simulink model "BothOptimizedNew"  (R2024b)
settings: Solver=FixedStepAuto  StartTime=0.0  StopTime=10.0  RelTol=1e-3  EnableMultiTasking=on
undefined symbols (not defined in the file or in its folder): samplingTime
settings Model: STM32="{\"DigitalPortWrite\":[{\"ID\":\"MicroMouseTemplate:84:3\"},{\"ID\":\"MicroMouseTemplate:84:4\"},{\"ID\":\"MicroMouseTemplate:84:5\"},{\"ID\":\"MicroMouseTemplate:84:6\"},{\"ID\":\"MicroMouseTemplate:84:7\"},{\"ID\":\"MicroMouseTemplate:84:8\"},{\"ID\":\"MicroMouseTemplate:84:9\"},{\"ID\":\"MicroMouseTemplate:84:10\"},{\"ID\":\"MicroMouseTemplate:160:19\"},{\"ID\":\"MicroMouseTemplate:2479:4\"},{\"ID\":\"MicroMouseTemplate:2479:6\"},{\"ID\":\"MicroMouseTemplate:2479:7\"},{\"ID\":\"MicroMouseTemplate:2479:8\"},{\"ID\":\"MicroMouseTemplate2:160:19\"},{\"ID\":\"MicroMouseTemplate2:2479:4\"},{\"ID\":\"MicroMouseTemplate2:2479:6\"},{\"ID\":\"MicroMouseTemplate2:2479:7\"},{\"ID\":\"MicroMouseTemplate2:2479:8\"},{\"ID\":\"MicroMouseTemplate2:84:3\"},{\"ID\":\"MicroMouseTemplate2:84:4\"},{\"ID\":\"MicroMouseTemplate2:84:5\"},{\"ID\":\"MicroMouseTemplate2:84:6\"},{\"ID\":\"MicroMouseTemplate2:84:7\"},{\"ID\":\"MicroMouseTemplate2:84:8\"},{\"ID\":\"MicroMouseTemplate2:84:9\"},{\"ID\":\"MicroMouseTemplate2:84:10\"},{\"ID\":\"MicroMouseTemplateTest:160:19\"},{\"ID\":\"MicroMouseTemplateTest:2479:4\"},{\"ID\":\"MicroMouseTemplateTest:2479:6\"},{\"ID\":\"MicroMouseTemplateTest:2479:7\"},{\"ID\":\"MicroMouseTemplateTest:2479:8\"},{\"ID\":\"MicroMouseTemplateTest:84:3\"},{\"ID\":\"MicroMouseTemplateTest:84:4\"},{\"ID\":\"MicroMouseTemplateTest:84:5\"},{\"ID\":\"MicroMouseTemplateTest:84:6\"},{\"ID\":\"MicroMouseTemplateTest:84:7\"},{\"ID\":\"MicroMouseTemplateTest:84:8\"},{\"ID\":\"MicroMouseTemplateTest:84:9\"},{\"ID\":\"MicroMouseTemplateTest:84:10\"},{\"ID\":\"MicroMouseTemplateTest2:160:19\"},{\"ID\":\"MicroMouseTemplateTest2:2479:4\"},{\"ID\":\"MicroMouseTemplateTest2:2479:6\"},{\"ID\":\"MicroMouseTemplateTest2:2479:7\"},{\"ID\":\"MicroMouseTemplateTest2:2479:8\"},{\"ID\":\"MicroMouseTemplateTest2:84:3\"},{\"ID\":\"MicroMouseTemplateTest2:84:4\"},{\"ID\":\"MicroMouseTemplateTest2:84:5\"},{\"ID\":\"MicroMouseTemplateTest2:84:6\"},{\"ID\":\"MicroMouseTemplateTest2:84:7\"},{\"ID\":\"MicroMouseTemplateTest2:84:8\"},{\"ID\":\"MicroMouseTemplateTest2:84:9\"},{\"ID\":\"MicroMouseTemplateTest2:84:10\"},{\"ID\":\"HalfOptimized:84:10\"},{\"ID\":\"HalfOptimized:84:9\"},{\"ID\":\"HalfOptimized:84:8\"},{\"ID\":\"HalfOptimized:84:7\"},{\"ID\":\"HalfOptimized:84:6\"},{\"ID\":\"HalfOptimized:84:5\"},{\"ID\":\"HalfOptimized:84:4\"},{\"ID\":\"HalfOptimized:84:3\"},{\"ID\":\"HalfOptimized:160:19\"},{\"ID\":\"HalfOptimized:2479:4\"},{\"ID\":\"HalfOptimized:2479:6\"},{\"ID\":\"HalfOptimized:2479:7\"},{\"ID\":\"HalfOptimized:2479:8\"},{\"ID\":\"HalfOptimized4:84:3\"},{\"ID\":\"HalfOptimized4:84:4\"},{\"ID\":\"HalfOptimized4:84:5\"},{\"ID\":\"HalfOptimized4:84:6\"},{\"ID\":\"HalfOptimized4:84:7\"},{\"ID\":\"HalfOptimized4:84:8\"},{\"ID\":\"HalfOptimized4:84:9\"},{\"ID\":\"HalfOptimized4:84:10\"},{\"ID\":\"HalfOptimized4:160:19\"},{\"ID\":\"HalfOptimized4:2479:4\"},{\"ID\":\"HalfOptimized4:2479:6\"},{\"ID\":\"HalfOptimized4:2479:7\"},{\"ID\":\"HalfOptimized4:2479:8\"},{\"ID\":\"LeftOptimized4:84:3\"},{\"ID\":\"LeftOptimized4:84:4\"},{\"ID\":\"LeftOptimized4:84:5\"},{\"ID\":\"LeftOptimized4:84:6\"},{\"ID\":\"LeftOptimized4:84:7\"},{\"ID\":\"LeftOptimized4:84:8\"},{\"ID\":\"LeftOptimized4:84:9\"},{\"ID\":\"LeftOptimized4:84:10\"},{\"ID\":\"LeftOptimized4:160:19\"},{\"ID\":\"LeftOptimized4:2479:4\"},{\"ID\":\"LeftOptimized4:2479:6\"},{\"ID\":\"LeftOptimized4:2479:7\"},{\"ID\":\"LeftOptimized4:2479:8\"},{\"ID\":\"BothOptimizedNew:84:3\"},{\"ID\":\"BothOptimizedNew:84:4\"},{\"ID\":\"BothOptimizedNew:84:5\"},{\"ID\":\"BothOptimizedNew:84:6\"},{\"ID\":\"BothOptimizedNew:84:7\"},{\"ID\":\"BothOptimizedNew:84:8\"},{\"ID\":\"BothOptimizedNew:84:9\"},{\"ID\":\"BothOptimizedNew:84:10\"},{\"ID\":\"BothOptimizedNew:160:19\"},{\"ID\":\"BothOptimizedNew:2479:4\"},{\"ID\":\"BothOptimizedNew:2479:6\"},{\"ID\":\"BothOptimizedNew:2479:7\"},{\"ID\":\"BothOptimizedNew:2479:8\"}],\"PWMOutput\":[{\"ID\":\"MicroMouseTemplate:160:24\"},{\"ID\":\"MicroMouseTemplate:160:25\"},{\"ID\":\"MicroMouseTemplate2:160:24\"},{\"ID\":\"MicroMouseTemplate2:160:25\"},{\"ID\":\"MicroMouseTemplateTest:160:24\"},{\"ID\":\"MicroMouseTemplateTest:160:25\"},{\"ID\":\"MicroMouseTemplateTest2:160:24\"},{\"ID\":\"MicroMouseTemplateTest2:160:25\"},{\"ID\":\"HalfOptimized:160:24\"},{\"ID\":\"HalfOptimized:160:25\"},{\"ID\":\"HalfOptimized4:160:24\"},{\"ID\":\"HalfOptimized4:160:25\"},{\"ID\":\"LeftOptimized4:160:24\"},{\"ID\":\"LeftOptimized4:160:25\"},{\"ID\":\"BothOptimizedNew:160:24\"},{\"ID\":\"BothOptimizedNew:160:25\"}],\"AnalogInput\":[{\"ID\":\"MicroMouseTemplate:2357:1\"},{\"ID\":\"MicroMouseTemplate2:2357:1\"},{\"ID\":\"MicroMouseTemplateTest:2357:1\"},{\"ID\":\"MicroMouseTemplateTest2:2357:1\"},{\"ID\":\"HalfOptimized:2357:1\"},{\"ID\":\"HalfOptimized4:2357:1\"},{\"ID\":\"LeftOptimized4:2357:1\"},{\"ID\":\"BothOptimizedNew:2357:1\"}],\"DigitalPortRead\":[{\"ID\":\"MicroMouseTemplate:2483:3\"},{\"ID\":\"MicroMouseTemplate:2483:4\"},{\"ID\":\"MicroMouseTemplate2:2483:3\"},{\"ID\":\"MicroMouseTemplate2:2483:4\"},{\"ID\":\"MicroMouseTemplateTest:2483:3\"},{\"ID\":\"MicroMouseTemplateTest:2483:4\"},{\"ID\":\"MicroMouseTemplateTest2:2483:3\"},{\"ID\":\"MicroMouseTemplateTest2:2483:4\"},{\"ID\":\"HalfOptimized:2483:3\"},{\"ID\":\"HalfOptimized:2483:4\"},{\"ID\":\"HalfOptimized4:2483:3\"},{\"ID\":\"HalfOptimized4:2483:4\"},{\"ID\":\"LeftOptimized4:2483:3\"},{\"ID\":\"LeftOptimized4:2483:4\"},{\"ID\":\"BothOptimizedNew:2483:3\"},{\"ID\":\"BothOptimizedNew:2483:4\"}]}"  SimulationMode=external  ExtModeTrigDuration=10  Creator=JesseJabezArendse  LastModifiedBy=Nang'alelwa
settings SolverCC: AllowMultiTaskInputOutput=on  AutoInsertRateTranBlk=on  InsertRTBMode=Never (minimum delay)
settings OptimizationCC: EnhancedBackFolding=on  PassReuseOutputArgsAs=Individual arguments  StateBitsets=on  DataBitsets=on  ZeroExternalMemoryAtStartup=off  ZeroInternalMemoryAtStartup=off  NoFixptDivByZeroProtection=on  MaxStackSize=64  OptimizeBlockOrder=speed  DifferentSizesBufferReuse=on  EfficientTunableParamExpr=on
settings DebuggingCC: MultiTaskCondExecSysMsg=none  ParameterOverflowMsg=none  ParameterPrecisionLossMsg=none  ParameterTunabilityLossMsg=error
settings HardwareCC: ProdBitPerPointer=32  ProdBitPerSizeT=32  ProdBitPerPtrDiffT=32  ProdLargestAtomicInteger=Long  ProdLargestAtomicFloat=Double  ProdWordSize=32  ProdLongLongMode=on  ProdHWDeviceType=ARM Compatible->ARM Cortex  TargetBitPerPointer=64  TargetBitPerSizeT=64  TargetBitPerPtrDiffT=64  TargetLongLongMode=on  TargetIntDivRoundTo=Zero  TargetEndianess=LittleEndian  TargetWordSize=64  TargetHWDeviceType=MATLAB Host
settings ModelReferenceCC: EnableParallelModelReferenceBuilds=on  ParallelModelReferenceMATLABWorkerInit=Copy Base Workspace  SupportModelReferenceSimTargetCustomCode=on
settings SFSimCC: MATLABDynamicMemAlloc=off  SimHardwareAcceleration=native
settings RTWCC: Description=Embedded Coder  SystemTargetFile=ert.tlc  HardwareBoard=STM32L4xx Based  TLCOptions=-p0 -aInlineSetEventsForThisBaseRateFcn=TLC_FALSE -aSuppressMultiTaskScheduler=TLC_FALSE -aRateBasedStepFcn=1  TemplateMakefile=ert_default_tmf  Toolchain=GNU Tools for ARM Embedded Processors  CodeExecutionProfiling=on  CodeProfilingInstrumentation=coarse  GPUComputeCapability=3.5
settings RTWCC: CustomHeaderCode=|
  | #include "MicroMouseProgramming\Core\Inc\IMU.h"
  | #include "MicroMouseProgramming\Core\Inc\CustomWhile.h"
  | #include "MicroMouseProgramming\Core\Inc\Motors.h"
settings RTWCC: CustomInclude=|
  | MicroMouseProgramming\Core\Inc\
  | MicroMouseProgramming\Core\Src\
settings RTWCC: CustomSource=|
  | MicroMouseProgramming\Core\Src\IMU.c
  | MicroMouseProgramming\Core\Src\CustomWhile.c
  | MicroMouseProgramming\Core\Src\Motors.c
settings CodeAppCC: ForceParamTrailComments=on  IgnoreCustomStorageClasses=off  OperatorAnnotations=on  SimulinkDataObjDesc=on  SFDataObjDesc=on  InsertBlockDesc=on
settings ERTTargetCC: CodeReplacementLibrary=ARM Cortex-M  SupportNonFinite=off  SupportComplex=off  ExtModeTransport=3  ExtModeStaticAlloc=on  ExtModeStaticAllocSize=2048  ExtModeMexFile=ext_xcp  ExtModeIntrfLevel=Level2 - Open  InlinedParameterPlacement=Hierarchical  DynamicArrayContainerType=coder::array

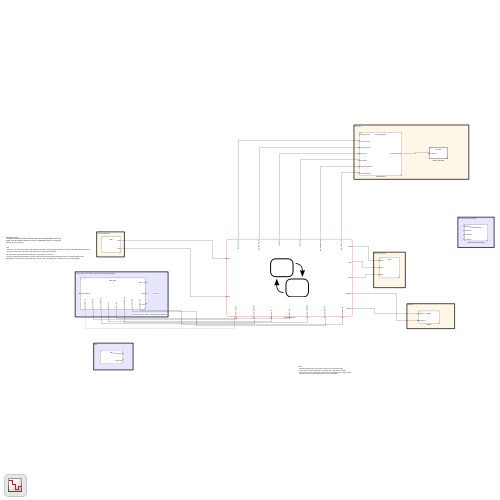
[thumbnail: Simulink's stored preview of the top-level diagram]
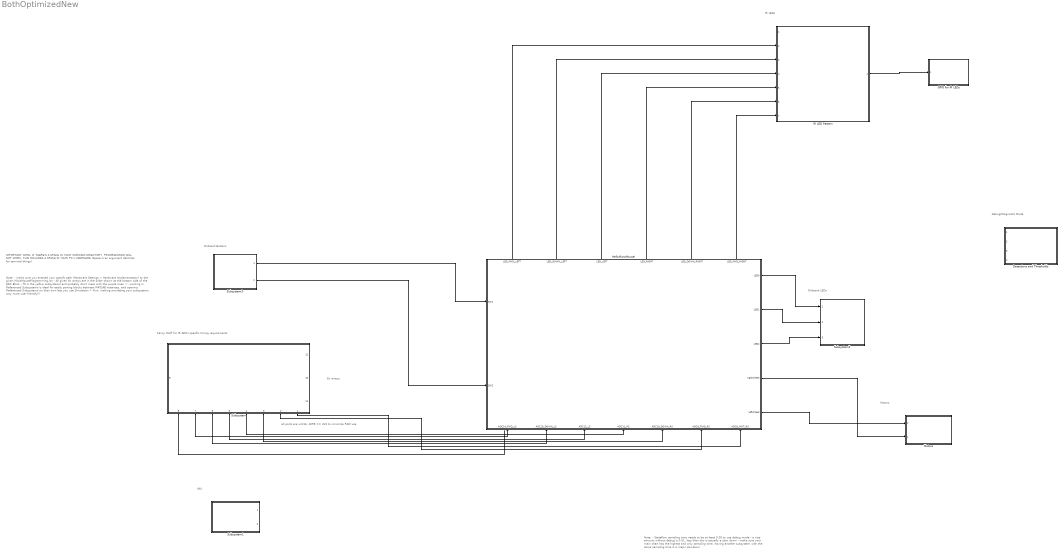
== system BothOptimizedNew ==
  note: IMPORTANT NOTE:
      | IF THERE'S A SPACE IN YOUR WORKING DIRECTORY, PROGRAMMING WILL NOT WORK, THIS INCLUDES A SPACE IN YOUR PC's USERNAME (Space is an argument delimiter for terminal things)
  note: Note:
      | - make sure you entered your specifc path (Hardware Settings > Hardware Implementation) to the given MicroMouseProgramming.ioc
      | - All given 8x arrays are in the order shown at the bottom side of the ADC Block
      |
      | - fill in the yellow subsystems and probably don't mess with the purple ones :)
      | - working in Referenced Subsystems is ideal for easily porting blocks between MATLAB instances, and opening Referenced Subsystems on their own lets you use Simulation > Run, making simulating your subsystems way more user friendly!!!
  note: 8x arrays
  note: all ports are uint16, 4095 == 3V3 to minimize RAM use
  note: IMU
  note: Note:
      | - Stateflow sampling time needs to be at least 0.05 to use debug mode
      | - a nice amount without debug is 0.01, less than this is actually a slow down
      | - make sure your main chart has the highest and only sampling time, having another
      | subsystem with the same sampling time is a major slowdown
  note: Fancy Stuff for IR ADCs specific timing requirements
  note: IR LEDs
  note: Motors
  note: Onboard Buttons
  note: Onboard LEDs
  note: Debug/Diagnostic Mode
  Detections and Thresholds : Subsystem  ReferencedSubsystem=DiagnosticMode
  GPIO for IR LEDs : Subsystem  TreatAsAtomicUnit=on  SystemSampleTime=samplingTime  ReferencedSubsystem=IR_LEDs
  HelloMicroMouse! : Stateflow chart  TreatAsAtomicUnit=on
      settings: PortSchema="{\"entries\":[{\"content\":{\"sides\":[{\"content\":{\"connectorIds\":[\"In9\",\"In8\"]},\"type\":\"ConnectorPlacement.EquallySpacedRectSide\",\"uuid\":\"f52daa4f-6374-42e5-9ef1-0ccc99d09b58\"},{\"content\":{\"connectorIds\":[\"Out11\",\"Out5\",\"Out6\",\"Out2\",\"Out1\"],\"side\":\"RIGHT\"},\"type\":\"ConnectorPlacement.EquallySpacedRectSide\",\"uuid\":\"94b478cc-4dde-45c7-a588-77cf2b43cdb7\"},{\"content\":{\"connectorIds\":[\"Out3\",\"Out4\",\"Out7\",\"Out8\",\"Out9\",\"Out10\"],\"side\":\"TOP\"},\"type\":\"ConnectorPlacement.EquallySpacedRectSide\",\"uuid\":\"afff2079-ea5c-423e-9722-09c3bbce433b\"},{\"content\":{\"connectorIds\":[\"In1\",\"In2\",\"In3\",\"In4\",\"In5\",\"In6\",\"In7\"],\"side\":\"BOTTOM\"},\"type\":\"ConnectorPlacement.EquallySpacedRectSide\",\"uuid\":\"94e93a1d-795d-41a3-b2d8-d520b2bf47ef\"}]},\"type\":\"ConnectorPlacement.EquallySpacedConnector\",\"uuid\":\"d4d35636-54af-48ac-af70-d56caef5e090\"}],\"packageUris\":[\"http://schema.mathworks.com/mf0/Connector/R2020b\"],\"version\":\"1.0\"}"
  IR LED Pattern : Subsystem  ReferencedSubsystem=IR_LED_Pattern
  Motors : Subsystem  ReferencedSubsystem=Motors
      settings: PortSchema="{\"entries\":[{\"content\":{\"sides\":[{\"content\":{\"connectorIds\":[\"In2\",\"In1\"]},\"type\":\"ConnectorPlacement.EquallySpacedRectSide\",\"uuid\":\"b3741f01-871a-479c-9206-f0581f668097\"},{\"content\":{\"side\":\"RIGHT\"},\"type\":\"ConnectorPlacement.EquallySpacedRectSide\",\"uuid\":\"4e24163a-f10e-40fa-a35f-86add3e4876d\"},{\"content\":{\"side\":\"TOP\"},\"type\":\"ConnectorPlacement.EquallySpacedRectSide\",\"uuid\":\"20b900cb-8f31-42f3-9ac1-0d679ccd8bc0\"}]},\"type\":\"ConnectorPlacement.EquallySpacedConnector\",\"uuid\":\"90358f46-f7a9-48cf-9149-c68081c17f53\"}],\"packageUris\":[\"http://schema.mathworks.com/mf0/Connector/R2020b\"],\"version\":\"1.0\"}"
  Subsystem : Subsystem  ReferencedSubsystem=ADC_Block
      settings: PortSchema="{\"entries\":[{\"content\":{\"sides\":[{\"content\":{},\"type\":\"ConnectorPlacement.EquallySpacedRectSide\",\"uuid\":\"be6b81d5-7a49-4e34-b35f-0c07892094fc\"},{\"content\":{\"connectorIds\":[\"Out1\",\"Out2\",\"Out3\",\"Out4\",\"Out5\",\"Out6\",\"Out7\",\"Out8\"],\"side\":\"RIGHT\"},\"type\":\"ConnectorPlacement.EquallySpacedRectSide\",\"uuid\":\"5e22590a-b7c0-4c63-8de4-8d81fd6c3849\"},{\"content\":{\"connectorIds\":[\"Out12\",\"Out10\",\"Out11\"],\"side\":\"TOP\"},\"type\":\"ConnectorPlacement.EquallySpacedRectSide\",\"uuid\":\"da97636e-cea0-4a10-8fe5-d807f9ee999f\"},{\"content\":{\"connectorIds\":[\"Out9\"],\"side\":\"BOTTOM\"},\"type\":\"ConnectorPlacement.EquallySpacedRectSide\",\"uuid\":\"a593d780-81a8-4730-a8bc-2bbf356cafe4\"}]},\"type\":\"ConnectorPlacement.EquallySpacedConnector\",\"uuid\":\"0bcac921-e51a-4437-9183-315712d0a8c2\"}],\"packageUris\":[\"http://schema.mathworks.com/mf0/Connector/R2020b\"],\"version\":\"1.0\"}"
  Subsystem1 : Subsystem  ReferencedSubsystem=IMU
  Subsystem2 : Subsystem  ReferencedSubsystem=LEDs
  Subsystem3 : Subsystem  ReferencedSubsystem=SWs
  wires:
  HelloMicroMouse!/2(rightWheel) -> Motors/1
  HelloMicroMouse!/1(leftWheel) -> Motors/2
  IR LED Pattern/1 -> GPIO for IR LEDs/1
  Subsystem3/1 -> HelloMicroMouse!/9(SW1)
  Subsystem3/2 -> HelloMicroMouse!/8(SW2)
  HelloMicroMouse!/11(LED0) -> Subsystem2/1
  Subsystem/8 -> ?
  Subsystem/7 -> HelloMicroMouse!/1(ADC14_FWD_LS)
  Subsystem/6 -> HelloMicroMouse!/2(ADC13_DOWN_LS)
  Subsystem/5 -> HelloMicroMouse!/3(ADC12_LS)
  Subsystem/4 -> HelloMicroMouse!/4(ADC11_RS)
  Subsystem/3 -> HelloMicroMouse!/5(ADC10_DOWN_RS)
  Subsystem/2 -> HelloMicroMouse!/6(ADC9_FWD_RS)
  Subsystem/1 -> HelloMicroMouse!/7(ADC8_MOT_RS)
  HelloMicroMouse!/5(LED1) -> Subsystem2/2
  HelloMicroMouse!/6(LED2) -> Subsystem2/3
  HelloMicroMouse!/10(LED_FWD_RIGHT) -> IR LED Pattern/7
  HelloMicroMouse!/9(LED_DOWN_RIGHT) -> IR LED Pattern/6
  HelloMicroMouse!/8(LED_RIGHT) -> IR LED Pattern/5
  HelloMicroMouse!/7(LED_LEFT) -> IR LED Pattern/4
  HelloMicroMouse!/4(LED_DOWN_LEFT) -> IR LED Pattern/3
  HelloMicroMouse!/3(LED_FWD_LEFT) -> IR LED Pattern/2

== stateflow chart BothOptimizedNew/HelloMicroMouse! ==
  state Turns1 [commented out]
    entry:
    solved = 0
    LED0 = false;
    LED1 = false;
    LED2 = false;
    R = 1;
    S = 2;
    L = 3;
    B = 4;
    stop = 0
    state TurnLeftToLeft1 [commented out]
      entry:
      leftWheel = -75;
      rightWheel = 75;
    state CheckLeftWall1 [commented out]
      entry:
      leftWheel = 0;
      rightWheel = 0;
      if (ADC14_FWD_LS >0.85* init_FWD_LEFT &&  ADC9_FWD_RS >0.85* init_FWD_RIGHT)
      LED1 = false;
      else
      SolvedAlgorithm(index) = L;
      index = index +1;
      stop = 1
      LED1 = true;
      end
    state MoveCentre [commented out]
      entry:
      leftWheel = 75;
      rightWheel = 75;
    state CheckStraightWall [commented out]
      entry:
      leftWheel = 0;
      rightWheel = 0;
      if (ADC14_FWD_LS >0.85* init_FWD_LEFT &&  ADC9_FWD_RS >0.8* init_FWD_RIGHT)
      LED1 = false;
      else
      SolvedAlgorithm(index) = S;
      index = index +1;
      stop = 1;
      LED1 = true;
      end
    state TurnRightToStraight [commented out]
      entry:
      leftWheel = 75;
      rightWheel = -75;
    state CheckLeftWall [commented out]
      entry:
      leftWheel = 0;
      rightWheel = 0;
      if (ADC14_FWD_LS >0.80* init_FWD_LEFT &&  ADC9_FWD_RS >0.85* init_FWD_RIGHT)
      LED1 = false;
      else
      SolvedAlgorithm(index) = R;
      index = index +1;
      stop = 1
      LED1 = true;
      end
    state TurnRightToRight [commented out]
      entry:
      leftWheel = 75;
      rightWheel = -75;
    state CheckWallBack [commented out]
      entry:
      leftWheel = 0;
      rightWheel = 0;
      during:
      if (ADC14_FWD_LS >0.85* init_FWD_LEFT &&  ADC9_FWD_RS >0.87* init_FWD_RIGHT)
      LED1 = false;
      else
      SolvedAlgorithm(index) = B;
      index = index +1;
      stop = 1
      LED1 = true;
      end
    state TurnLeftToBack [commented out]
      entry:
      leftWheel = 75;
      rightWheel = -75;
    (default) -> Turns1.MoveCentre [commented out]
    Turns1.CheckWallBack -> TurnLeftToLeft1 [commented out] : [SW2]
    TurnLeftToLeft1 -> CheckLeftWall1 [commented out] : after(1.2, sec)
    Turns1.MoveCentre -> TurnLeftToLeft1 [commented out] : after(0.4,sec)
    CheckLeftWall1 -> TurnRightToStraight [commented out] : after(1.2,sec)
    TurnRightToStraight -> Turns1.CheckStraightWall [commented out] : after(1.2,sec)
    Turns1.CheckStraightWall -> Turns1.TurnRightToRight [commented out] : after(1.1,sec)
    Turns1.TurnRightToRight -> Turns1.CheckLeftWall [commented out] : after(1.2,sec)
    Turns1.CheckLeftWall -> Turns1.TurnLeftToBack [commented out] : after(1.2,sec)
    Turns1.TurnLeftToBack -> Turns1.CheckWallBack [commented out] : after(1.2 ,sec)
  state Turns
    entry:
    solved = 0
    LED0 = false;
    LED1 = false;
    LED2 = false;
    R = 1;
    S = 2;
    L = 3;
    B = 4;
    state TurnRightToRight
      entry:
      leftWheel = 75;
      rightWheel = -75;
    state CheckRightWall
      entry:
      leftWheel = 0;
      rightWheel = 0;
      if (ADC14_FWD_LS >0.8* init_FWD_LEFT &&  ADC9_FWD_RS >0.8* init_FWD_RIGHT)
      LED1 = false;
      else
      SolvedAlgorithm(index) = R;
      index = index +1;
      LED1 = true;
      end
    state MoveCentre
      entry:
      leftWheel = 75;
      rightWheel = 75;
    state CheckStraightWall
      entry:
      leftWheel = 0;
      rightWheel = 0;
      if (ADC14_FWD_LS >0.8* init_FWD_LEFT &&  ADC9_FWD_RS >0.8* init_FWD_RIGHT)
      LED1 = false;
      else
      SolvedAlgorithm(index) = S;
      index = index +1;
      LED1 = true;
      end
    state TurnLeftToStraight
      entry:
      leftWheel = -75;
      rightWheel = 75;
    state CheckLeftWall
      entry:
      leftWheel = 0;
      rightWheel = 0;
      if (ADC14_FWD_LS >0.8* init_FWD_LEFT &&  ADC9_FWD_RS >0.8* init_FWD_RIGHT)
      LED1 = false;
      else
      SolvedAlgorithm(index) = L;
      index = index +1;
      LED1 = true;
      end
    state TurnLeftToLeft
      entry:
      leftWheel = -75;
      rightWheel = 75;
    state CheckWallBack
      entry:
      leftWheel = 0;
      rightWheel = 0;
      during:
      if (ADC14_FWD_LS >0.8* init_FWD_LEFT &&  ADC9_FWD_RS >0.8* init_FWD_RIGHT)
      LED1 = false;
      else
      SolvedAlgorithm(index) = B;
      index = index +1;
      LED1 = true;
      end
    state TurnLeftToBack
      entry:
      leftWheel = -75;
      rightWheel = 75;
    (default) -> Turns.MoveCentre
    Turns.CheckWallBack -> Turns.TurnRightToRight : [SW2]
    Turns.TurnRightToRight -> CheckRightWall : after(1.1, sec)
    Turns.MoveCentre -> Turns.TurnRightToRight : after(0.4,sec)
    CheckRightWall -> TurnLeftToStraight : after(1.1,sec)
    TurnLeftToStraight -> Turns.CheckStraightWall : after(1.2,sec)
    Turns.CheckStraightWall -> TurnLeftToLeft : after(1.1,sec)
    TurnLeftToLeft -> Turns.CheckLeftWall : after(1.2,sec)
    Turns.CheckLeftWall -> Turns.TurnLeftToBack : after(1.1,sec)
    Turns.TurnLeftToBack -> Turns.CheckWallBack : after(1.2 ,sec)
  state Placeholder2
    entry:
    index = 1;
    leftWheel = 0;
    rightWheel = 0;
    solved = 1;
    optimisedPath =optimize_path(SolvedAlgorithm);
    during:
    LED1=~LED1;
  state Calibration_Forward1
    entry:
    LED0 = false;
    LED1 = true;
    LED2 = false
    LED_LEFT = false;
    LED_RIGHT = false;
    LED_FWD_LEFT = true;
    LED_FWD_RIGHT = true;
    LED_DOWN_RIGHT = true;
    LED_DOWN_LEFT = true;
    counter = 0
    sum_FWD_LEFT = 0;
    sum_FWD_RIGHT = 0;
    during:
    if counter < 8000
    sum_FWD_LEFT = sum_FWD_LEFT + ADC14_FWD_LS;
    sum_FWD_RIGHT = sum_FWD_RIGHT + ADC9_FWD_RS;
    counter = counter + 1;
    end
    exit:
    avg_FWD_LEFT = sum_FWD_LEFT / counter;
    avg_FWD_RIGHT = sum_FWD_RIGHT / counter;
    init_FWD_LEFT = avg_FWD_LEFT;
    init_FWD_RIGHT = avg_FWD_RIGHT;
    LED1 = false
  state LineFollowing
    entry:
    LED0 = false;
    LED1 = false;
    LED2 = false;
    LED_LEFT = false;
    LED_RIGHT = false;
    LED_FWD_LEFT = true;
    LED_FWD_RIGHT = true;
    LED_DOWN_RIGHT = true;
    LED_DOWN_LEFT = true;
    exit:
    LED0 = false;
    LED1 = false;
    LED2 = false;
    state Forward
      entry:
      LED1 = true;
      leftWheel = 80;
      rightWheel = 80;
      exit:
      LED1 = false;
    state Turning_Right_Adjustment
      entry:
      LED2 = true;
      leftWheel = 80;
      rightWheel = 70;
      exit:
      leftWheel = 0;
      LED2 = false;
    state Turning_Left_Adjustment
      entry:
      LED0 = true;
      rightWheel = 80;
      leftWheel = 70;
      exit:
      rightWheel = 0;
      LED0 = false;
    (default) -> LineFollowing.Forward
    LineFollowing.Forward -> Turning_Right_Adjustment [order 1] : [(ADC10_DOWN_RS >ADC13_DOWN_LS )  ]
    Turning_Right_Adjustment -> LineFollowing.Forward
    LineFollowing.Forward -> Turning_Left_Adjustment [order 2] : [(ADC10_DOWN_RS < ADC13_DOWN_LS ) ]
    Turning_Left_Adjustment -> LineFollowing.Forward
  state Calibration_Left_and_Right
    entry:
    LED0 = true;
    LED1 = false;
    LED2 = false
    LED_LEFT = true;
    LED_RIGHT = true;
    LED_FWD_LEFT = false;
    LED_FWD_RIGHT = false;
    LED_DOWN_RIGHT = false;
    LED_DOWN_LEFT = false;
    counter2 = 0
    sum_LEFT = 0;
    sum_RIGHT = 0;
    during:
    if counter2 < 8000
    sum_LEFT = sum_LEFT + ADC12_LS;
    sum_RIGHT = sum_RIGHT + ADC11_RS;
    counter2 = counter2 + 1;
    end
    exit:
    % Once 10 samples are collected, calculate the average
    avg_LEFT = sum_LEFT / counter2;
    avg_RIGHT = sum_RIGHT / counter2;
    % Use the averages for calibration or further processing
    init_LEFT = avg_LEFT;
    init_RIGHT = avg_RIGHT;
    end
    exit:
    LED0 = false
  state CrossRoad
    entry:
    LED0 = false;
    LED1 = false;
    LED2 = false;
    leftWheel = 0;
    rightWheel = 0;
    %during:
    %if (ADC14_FWD_LS >0.8* init_FWD_LEFT &&  ADC9_FWD_RS >0.8* init_FWD_RIGHT)
    %   LED1 = true;
    %else
    %    LED1 = false
    %end
    %LED_DOWN_RIGHT = false;
    %LED_DOWN_LEFT = false;
    %LED_FWD_LEFT = false;
    %LED_FWD_RIGHT = false;
    %LED_LEFT = true;
    %LED_RIGHT = true;
    %during:
    %if ADC12_LS > 0.85*init_LEFT
    %    LED2 = true;
    %else
    %   LED2 = false;
    %end
    %if ADC11_RS >0.85* init_RIGHT
    %LED0 = true;
    %else
    %    LED0 = false;
    %end
    %LED_LEFT = true;
    %LED_RIGHT = true;
    %LED_FWD_LEFT = false;
    %LED_FWD_RIGHT = false;
    %LED1 = ~LED1;
    %f ADC12_LS < 0.7* init_LEFT
    %    LED0 = true
    %end
    %if ADC11_RS < 0.7* init_RIGHT
    % LED2 = true
    %end
  state Calibration_Down1
    entry:
    LED2 = true
    LED_LEFT = false;
    LED_RIGHT = false;
    LED_FWD_LEFT = true;
    LED_FWD_RIGHT = true;
    LED_DOWN_RIGHT = true;
    LED_DOWN_LEFT = true;
    rightWheel = 75;
    leftWheel = -75;
    DOWN_R_DARK = ADC10_DOWN_RS;
    DOWN_L_DARK = ADC13_DOWN_LS;
    DOWN_R_LIGHT = ADC10_DOWN_RS;
    DOWN_L_LIGHT = ADC13_DOWN_LS;
    during:
    DOWN_R_DARK = min(DOWN_R_DARK, ADC10_DOWN_RS);
    DOWN_L_DARK = min(DOWN_L_DARK, ADC13_DOWN_LS);
    DOWN_R_LIGHT = max(DOWN_R_LIGHT, ADC10_DOWN_RS);
    DOWN_L_LIGHT = max(DOWN_L_LIGHT, ADC13_DOWN_LS);
  state WaitUntilButtonPressed6
    entry:
    LED_MOT_LEFT = false;
    LED_MOT_RIGHT = false;
    LED_FWD_LEFT = false;
    LED_FWD_RIGHT = false;
    LED_LEFT = false;
    LED_RIGHT = false;
    LED_DOWN_RIGHT = false;
    LED_DOWN_LEFT = false;
    during:
    LED1 = ~LED1;
  state Ready2
    entry:
    rightWheel = 0;
    leftWheel = 0;
    LED2 = true;
    LED0 = true;
    LED1 = true;
    maze = [
    0 1 0 0 0 1 0;
    0 1 0 1 0 1 0;
    0 0 0 1 0 0 0;
    1 1 0 0 0 1 1;
    0 0 0 1 0 0 0;
    0 1 0 1 0 1 0;
    0 0 0 0 0 0 0
    ];
    % Update flood fill matrix for a 7x7 grid
    flood = [6, 5, 4, 3, 4, 5, 6;
    5, 4, 3, 2, 3, 4, 5;
    4, 3, 2, 1, 2, 3, 4;
    3, 2, 1, 0, 1, 2, 3;  % Target cell is [4, 4] with flood value 0
    4, 3, 2, 1, 2, 3, 4;
    5, 4, 3, 2, 3, 4, 5;
    6, 5, 4, 3, 4, 5, 6];
    thresh_DOWN_RIGHT = (DOWN_R_LIGHT + DOWN_R_DARK)*0.5;
    thresh_DOWN_LEFT = (DOWN_L_LIGHT + DOWN_L_DARK)*0.5;
    SolvedAlgorithm = zeros(1, 100); % Predefine the array size
    index = 1;
  state Optimised
    entry:
    LED0 = true;
    LED1 = true;
    LED2 = true;
    next = 0;
    state Done1
      entry:
      leftWheel = 0;
      rightWheel = 0;
    state Checks
      entry:
      checking = optimisedPath(index);
      exit:
      index = index+1;
    state Forward
      entry:
      leftWheel = 0;
      rightWheel = 0;
      next =1
    state TurnRight
      entry:
      leftWheel = 75;
      rightWheel = 75;
    state TurnRight2
      entry:
      leftWheel = 75;
      rightWheel = -75;
    state TurnRight3
      entry:
      leftWheel = 0;
      rightWheel = 0;
      next = 1;
    state TurnAround
      entry:
      leftWheel = 75;
      rightWheel = -75;
    state TurnAround2
      entry:
      leftWheel = 0;
      rightWheel = 0;
      next = 1;
    state TurnLeft
      entry:
      leftWheel = 75;
      rightWheel = 75;
    state TurnLeft2
      entry:
      leftWheel = -75;
      rightWheel = 75;
    state TurnLeft3
      entry:
      leftWheel = 0;
      rightWheel = 0;
      next = 1;
    Checks -> Done1 [order 5] : [checking==0]
    (default) -> Checks
    Checks -> Optimised.Forward [order 2] : [checking == S]
    Checks -> TurnRight [order 1] : [checking == R]
    TurnRight2 -> TurnRight3 : after(1.1, sec)
    TurnRight -> TurnRight2 : after(0.4,sec)
    Checks -> TurnAround [order 3] : [checking == B]
    TurnAround -> TurnAround2 : after (2.3,sec)
    Checks -> TurnLeft [order 4] : [checking == L]
    TurnLeft -> TurnLeft2 : after(0.4,sec)
    TurnLeft2 -> TurnLeft3 : after(1.2,sec)
  Turns1 -> Placeholder2 [commented out] : [SW1]
  CrossRoad -> Turns1 [commented out] : [solved == 0 && after(1,sec)]
  Turns1 -> LineFollowing [commented out] : [LED1==true]
  Turns -> Placeholder2 [order 2] : [SW1]
  Turns -> LineFollowing [order 1] : [LED1 ==true]
  CrossRoad -> Turns [order 2] : [solved == 0 && after(1,sec)]
  Placeholder2 -> LineFollowing : [SW2]
  LineFollowing -> Placeholder2 [order 2] : [SW1]
  (default) -> WaitUntilButtonPressed6
  WaitUntilButtonPressed6 -> Calibration_Left_and_Right : [SW1]
  Calibration_Left_and_Right -> Calibration_Forward1 : [SW2]
  Calibration_Forward1 -> Calibration_Down1 : [SW1]
  Calibration_Down1 -> Ready2 : after(5, sec)
  Ready2 -> LineFollowing : [SW1]
  LineFollowing -> CrossRoad [order 1] : [ADC13_DOWN_LS < DOWN_L_DARK &&  ADC10_DOWN_RS < DOWN_R_DARK && after(1,sec)]
  CrossRoad -> LineFollowing [order 1] : [SW2]
  Optimised -> LineFollowing : [next==1]
  CrossRoad -> Optimised [order 3] : [solved == 1 && after(1,sec)]
  data: input_path function_input; optimized_path function_output; ADC14_FWD_LS input; ADC13_DOWN_LS input; ADC12_LS input; ADC11_RS input; ADC10_DOWN_RS input; ADC9_FWD_RS input; ADC8_MOT_RS input; leftWheel output; rightWheel output; LED_FWD_LEFT output; LED_DOWN_LEFT output; LED1 output =false; LED2 output =false; LED_LEFT output; LED_RIGHT output; LED_DOWN_RIGHT output; LED_FWD_RIGHT output; SW2 input; LED0 output =false; SW1 input; init_FWD_RIGHT local; init_FWD_LEFT local; DOWN_L_LIGHT local; thresh_DOWN_LEFT local; normal_speed_RIGHT local; DOWN_R_DARK local; DOWN_L_DARK local; thresh_DOWN_RIGHT local; DOWN_R_LIGHT local; normal_speed_LEFT local; avg_FWD_LEFT local; counter local; avg_FWD_RIGHT local; sum_FWD_LEFT local uint16; sum_FWD_RIGHT local uint16; avg_LEFT local; avg_RIGHT local; init_LEFT local; init_RIGHT local; sum_LEFT local uint16; sum_RIGHT local uint16; timer local; dark_val_l local; fwd_count local; light_val_r local; dark_val_r local; light_val_l local; lr_count local; motor_speed_left local; motor_speed_right local; thresh_LEFT local; thresh_RIGHT local; thresh_down_l local; thresh_down_r local; averageDown local; averageFront local; crossThreshold local; frontThreshold local; LED_MOT_LEFT local; LED_MOT_RIGHT local; flag local; counter2 local; R local; SolvedAlgorithm local; B local; checking local; index local; L local; next local; solved local; S local; flood local; ADC15_MOT_LS local; maze local; stop local; optimisedPath local
  function optimized_path = optimize_path(input_path):
    | function optimized_path = optimize_path(input_path)
    |     % This function takes a 1D array of integers as input and applies
    |     % optimization rules repeatedly until no further optimizations can be applied.
    |     
    |     % input_path is a 1D array of integers: 1=R, 2=S, 3=L, 4=B
    |     % optimized_path will be the same 1D array after applying rules, filled with zeros initially
    |     
    |     % Initial setup
    |     previous_path = input_path; 
    |     optimized_path = zeros(size(input_path)); % Preallocate the optimized path
    |     
    |     % Keep applying optimization until the path no longer changes
    |     while true
    |         % Index for the optimized path
    |         opt_index = 1;
    |         i = 1;
    |         
    |         % Traverse the path and apply the replacement rules
    |         while i <= length(previous_path)
    |             % Check if there are enough elements left to apply a rule (3 elements)
    |             if i <= length(previous_path) - 2
    |                 % Check for LBR -> B (3 4 1 -> 4)
    |                 if isequal(previous_path(i:i+2), [3, 4, 1])
    |                     optimized_path(opt_index) = 4;  % Replace with B
    |                     i = i + 3;  % Move forward by 3 elements in the input path
    |                 % Check for RBL -> B (1 4 3 -> 4)
    |                 elseif isequal(previous_path(i:i+2), [1, 4, 3])
    |                     optimized_path(opt_index) = 4;  % Replace with B
    |                     i = i + 3;
    |                 % Check for SBS -> B (2 4 2 -> 4)
    |                 elseif isequal(previous_path(i:i+2), [2, 4, 2])
    |                     optimized_path(opt_index) = 4;  % Replace with B
    |                     i = i + 3;
    |                 % Check for RBS -> L (1 4 2 -> 3)
    |                 elseif isequal(previous_path(i:i+2), [1, 4, 2])
    |                     optimized_path(opt_index) = 3;  % Replace with L
    |                     i = i + 3;
    |                 % Check for SBR -> L (2 4 1 -> 3)
    |                 elseif isequal(previous_path(i:i+2), [2, 4, 1])
    |                     optimized_path(opt_index) = 3;  % Replace with L
    |                     i = i + 3;
    |                 % Check for LBL -> S (3 4 3 -> 2)
    |                 elseif isequal(previous_path(i:i+2), [3, 4, 3])
    |                     optimized_path(opt_index) = 2;  % Replace with S
    |                     i = i + 3;
    |                 % Check for RBR -> S (1 4 1 -> 2)
    |                 elseif isequal(previous_path(i:i+2), [1, 4, 1])
    |                     optimized_path(opt_index) = 2;  % Replace with S
    |                     i = i + 3;
    |                 else
    |                     % If no rule is applied, just copy the current element
    |                     optimized_path(opt_index) = previous_path(i);
    |                     i = i + 1;  % Move to the next element in input path
    |                 end
    |             else
    |                 % For the last 2 or fewer elements, just copy them directly
    |                 optimized_path(opt_index) = previous_path(i);
    |                 i = i + 1;  % Move to the next element in input path
    |             end
    |             
    |             % Increment the index for the optimized path
    |             opt_index = opt_index + 1;
    |         end
    |         
    |         % If no changes were made, break the loop
    |         if isequal(previous_path, optimized_path)
    |             break;
    |         end
    |         
    |         % Update previous_path for the next iteration
    |         previous_path = optimized_path;
    |         optimized_path = zeros(size(previous_path)); % Reset optimized path
    |     end
    | end
